simulink model "Pendulum_Simulink"  (R2023a)
settings: Solver=VariableStepAuto  StartTime=0.0  StopTime=10.0  RelTol=1e-3
undefined symbols (not defined in the file): b, g, J, L, m, theta, theta_dot
settings Model: Creator=m260477  LastModifiedBy=m260477
settings DataIOCC: Refine=10

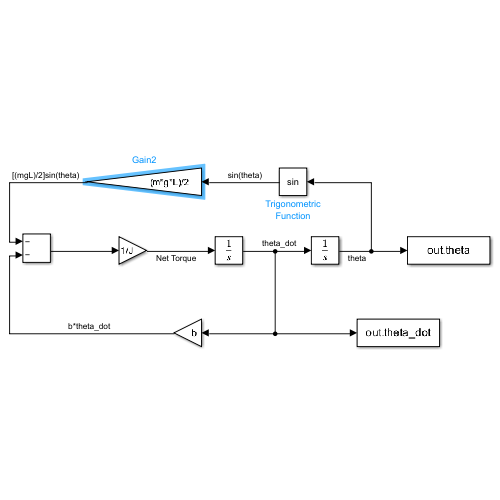
[thumbnail: Simulink's stored preview of the top-level diagram]
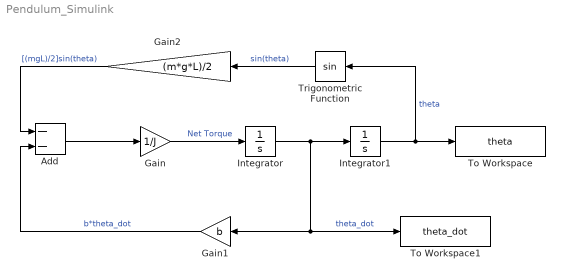
== system Pendulum_Simulink ==
  Add : Sum  Inputs=--
  Gain : Gain  Gain=1/J
  Gain1 : Gain  Gain=b
  Gain2 : Gain  Gain=(m*g*L)/2
  Integrator : Integrator  InitialCondition=theta_dot
  Integrator1 : Integrator  InitialCondition=theta
  To Workspace : ToWorkspace  VariableName=theta  SaveFormat=Timeseries  SampleTime=-1
  To Workspace1 : ToWorkspace  VariableName=theta_dot  SaveFormat=Timeseries  SampleTime=-1
  Trigonometric Function : Trigonometry
  wires:
  Add/1 -> Gain/1
  Gain/1 -> Integrator/1  "Net Torque"
  Integrator/1 -> To Workspace1/1, Gain1/1, Integrator1/1  "theta_dot"
  Integrator1/1 -> Trigonometric Function/1, To Workspace/1  "theta"
  Gain1/1 -> Add/2  "b*theta_dot"
  Trigonometric Function/1 -> Gain2/1  "sin(theta)"
  Gain2/1 -> Add/1  "[(mgL)/2]sin(theta)"
